simulink model "solar_pump_model"  (R2024b)
settings: Solver=VariableStepAuto  StartTime=0.0  StopTime=100  FixedStep=1  RelTol=1e-3
settings Model: LastModifiedBy=lerat

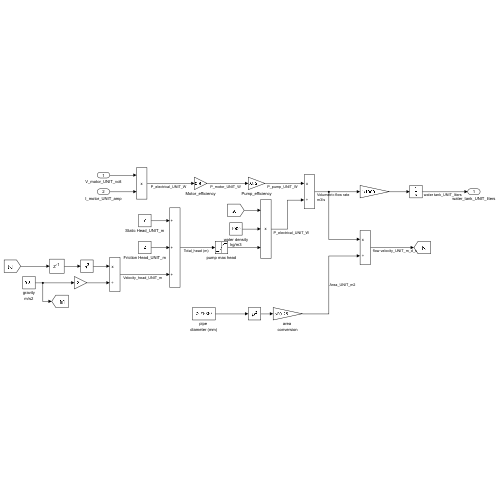
[thumbnail: Simulink's stored preview of the top-level diagram]
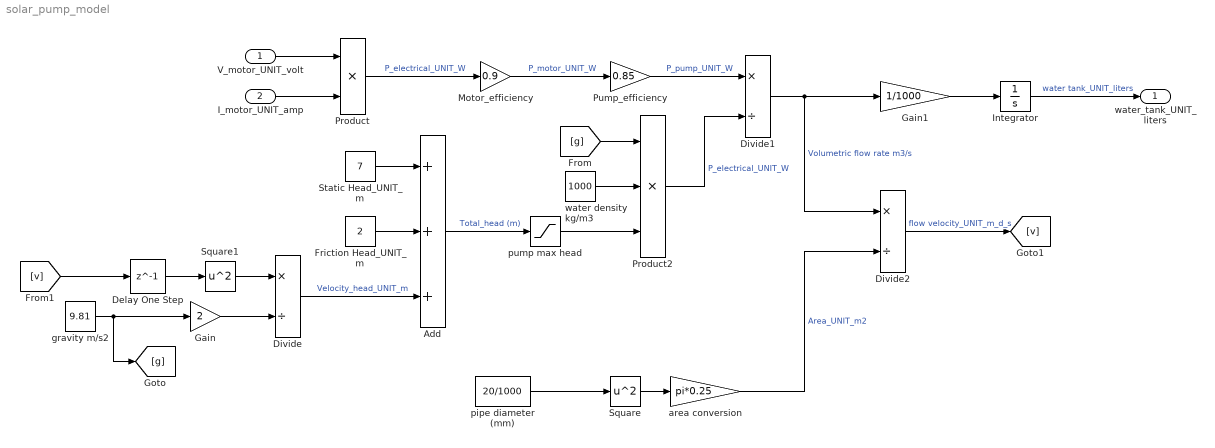
== system solar_pump_model ==
  V_motor_UNIT_volt : Inport
  I_motor_UNIT_amp : Inport  Port=2
  Add : Sum  Inputs=+++
  Delay One Step : Delay  DelayLength=1
  Divide : Product  Inputs=*/
  Divide1 : Product  Inputs=*/
  Divide2 : Product  Inputs=*/
  Friction Head_UNIT_m : Constant  Value=2
  Gain : Gain  Gain=2
  Gain1 : Gain  Gain=1/1000
  Integrator : Integrator
  Motor_efficiency : Gain  Gain=0.9
  Product : Product
  Product2 : Product  Inputs=3
  Pump_efficiency : Gain  Gain=0.85
  Square : Math  Operator=square
  Square1 : Math  Operator=square
  Static Head_UNIT_m : Constant  Value=7
  area conversion : Gain  Gain=pi*0.25
  gravity m/s2 : Constant  Value=9.81
  pipe diameter (mm) : Constant  Value=20/1000
  pump max head : Saturate  UpperLimit=9  LowerLimit=0
  water density kg/m3 : Constant  Value=1000
  water_tank_UNIT_liters : Outport
  wires:
  I_motor_UNIT_amp/1 -> Product/2
  V_motor_UNIT_volt/1 -> Product/1
  Product/1 -> Motor_efficiency/1  "P_electrical_UNIT_W"
  Motor_efficiency/1 -> Pump_efficiency/1  "P_motor_UNIT_W"
  Integrator/1 -> water_tank_UNIT_liters/1  "water tank_UNIT_liters"
  pipe diameter (mm)/1 -> Square/1
  Square/1 -> area conversion/1
  area conversion/1 -> Divide2/2  "Area_UNIT_m2"
  gravity m/s2/1 -> [g], Gain/1
  Square1/1 -> Divide/1
  Gain/1 -> Divide/2
  Divide/1 -> Add/3  "Velocity_head_UNIT_m"
  Static Head_UNIT_m/1 -> Add/1
  Friction Head_UNIT_m/1 -> Add/2
  Pump_efficiency/1 -> Divide1/1  "P_pump_UNIT_W"
  [g] -> Product2/1
  water density kg/m3/1 -> Product2/2
  Add/1 -> pump max head/1  "Total_head (m)"
  Product2/1 -> Divide1/2  "P_electrical_UNIT_W"
  Divide1/1 -> Gain1/1, Divide2/1  "Volumetric flow rate m3/s"
  Gain1/1 -> Integrator/1
  Divide2/1 -> [v]  "flow velocity_UNIT_m_d_s"
  Delay One Step/1 -> Square1/1
  [v] -> Delay One Step/1
  pump max head/1 -> Product2/3
